simulink model "Point_3"  (R2024b)
settings: Solver=VariableStepAuto  StartTime=0.0  StopTime=10.0  RelTol=1e-3
values from neighbouring files (symbols this model uses):
  Kd = (2*delta*omega_n+(-lambda3)-10)/(120)    [Script.m]
  Ki = (omega_n^2*(-lambda3))/(120)    (= 36)    [Script.m]
  Kp = (omega_n^2+2*delta*omega_n*(-lambda3))/(120)    [Script.m]
  Tl = 1/(8 * omega_n)    (= 0.0104166666667)    [Script.m]
undefined symbols (not defined in the file or in its folder): G
settings Model: Creator=farin  LastModifiedBy=farin

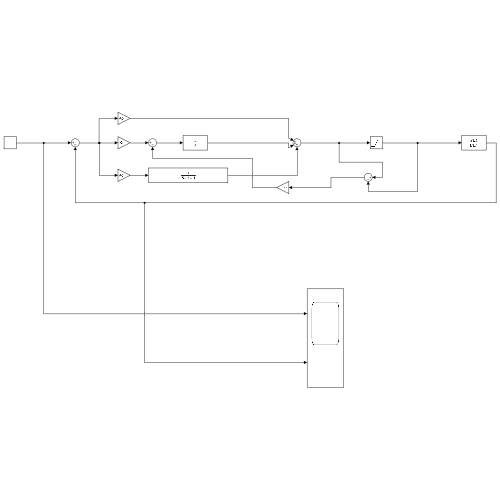
[thumbnail: Simulink's stored preview of the top-level diagram]
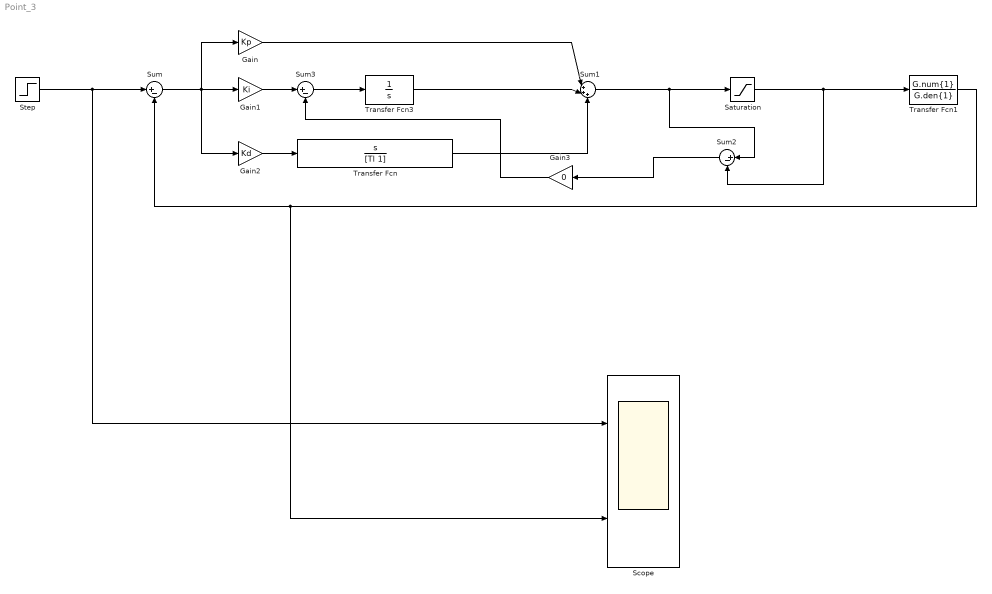
== system Point_3 ==
  Gain : Gain  Gain=Kp
  Gain1 : Gain  Gain=Ki
  Gain2 : Gain  Gain=Kd
  Gain3 : Gain  Gain=0
  Saturation : Saturate  UpperLimit=10  LowerLimit=-10
  Scope : Scope  NumInputPorts=2
  Step : Step  After=50  SampleTime=0
  Sum : Sum  Inputs=|+-
  Sum1 : Sum  Inputs=|+++
  Sum2 : Sum  Inputs=|+-
  Sum3 : Sum  Inputs=|+-
  Transfer Fcn : TransferFcn  Numerator=[1 0]  Denominator=[Tl 1]
  Transfer Fcn1 : TransferFcn  Numerator=G.num{1}  Denominator=G.den{1}
  Transfer Fcn3 : TransferFcn  Denominator=[1 0]
  wires:
  Transfer Fcn1/1 -> Scope/2, Sum/2
  Step/1 -> Scope/1, Sum/1
  Saturation/1 -> Sum2/2, Transfer Fcn1/1
  Sum/1 -> Gain2/1, Gain1/1, Gain/1
  Transfer Fcn/1 -> Sum1/3
  Transfer Fcn3/1 -> Sum1/2
  Gain/1 -> Sum1/1
  Sum1/1 -> Sum2/1, Saturation/1
  Sum2/1 -> Gain3/1
  Gain1/1 -> Sum3/1
  Gain3/1 -> Sum3/2
  Gain2/1 -> Transfer Fcn/1
  Sum3/1 -> Transfer Fcn3/1
